simulink model "testing"  (R2022b)
settings: Solver=VariableStepAuto  StartTime=0.0  StopTime=10.0  RelTol=1e-3
values from neighbouring files (symbols this model uses):
  A = 2    [scattering_params.m]    (also in scattering_params_force_pos.m = 3; scattering_params_pos_pos.m = 1)
  b = 1    [scattering_params.m]    (also in scattering_params_force_pos.m = 40; scattering_params_pos_pos.m = 100)
  Be = 100    [scattering_params.m]    (also in scattering_params_force_pos.m; scattering_params_pos_pos.m)
  Bh = 1.5    [scattering_params.m]    (also in scattering_params_force_pos.m = 1; scattering_params_pos_pos.m = 1)
  Bm = 20*0.8    (= 16)    [scattering_params.m]
  Bs = 80    [scattering_params.m]    (also in scattering_params_force_pos.m = 10)
  Dh = 0.1    [scattering_params.m]    (also in scattering_params_force_pos.m = 16; scattering_params_pos_pos.m = 16)
  Fc = 1    [scattering_params.m]    (also in scattering_params_force_pos.m = 0.25; scattering_params_pos_pos.m = 0.25)
  Flp = 5    [scattering_params.m]    (also in scattering_params_force_pos.m = 0.5; scattering_params_pos_pos.m = 0.5)
  Jh = 1    [scattering_params.m]    (also in scattering_params_force_pos.m; scattering_params_pos_pos.m)
  Ke = 200    [scattering_params.m]    (also in scattering_params_force_pos.m; scattering_params_pos_pos.m)
  Km = 10*1    (= 10)    [scattering_params.m]
  Ks = 100    [scattering_params.m]    (also in scattering_params_force_pos.m)
  Mm = 0.5    [scattering_params.m]    (also in scattering_params_force_pos.m; scattering_params_pos_pos.m)
  Ms = 2    [scattering_params.m]    (also in scattering_params_force_pos.m; scattering_params_pos_pos.m)
  Ph = 10    [scattering_params.m]    (also in scattering_params_force_pos.m; scattering_params_pos_pos.m)
  scattering_filter_freq = 10    [scattering_params.m]    (also in scattering_params_force_pos.m; scattering_params_pos_pos.m = 100)
  time_delay = 0    [scattering_params.m]
  xe = 5    [scattering_params.m]    (also in scattering_params_force_pos.m = 2; scattering_params_pos_pos.m = 2)
settings Model: Creator=Manu  LastModifiedBy=Manu

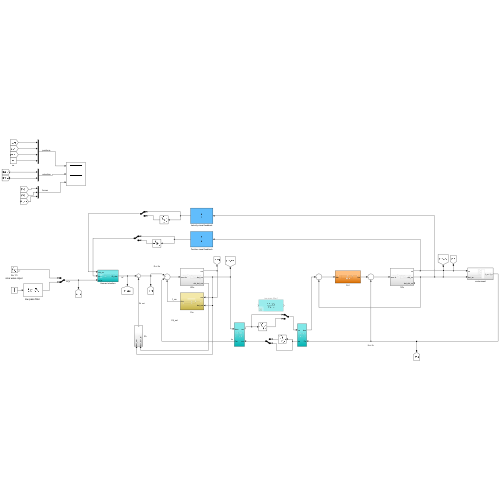
[thumbnail: Simulink's stored preview of the top-level diagram]
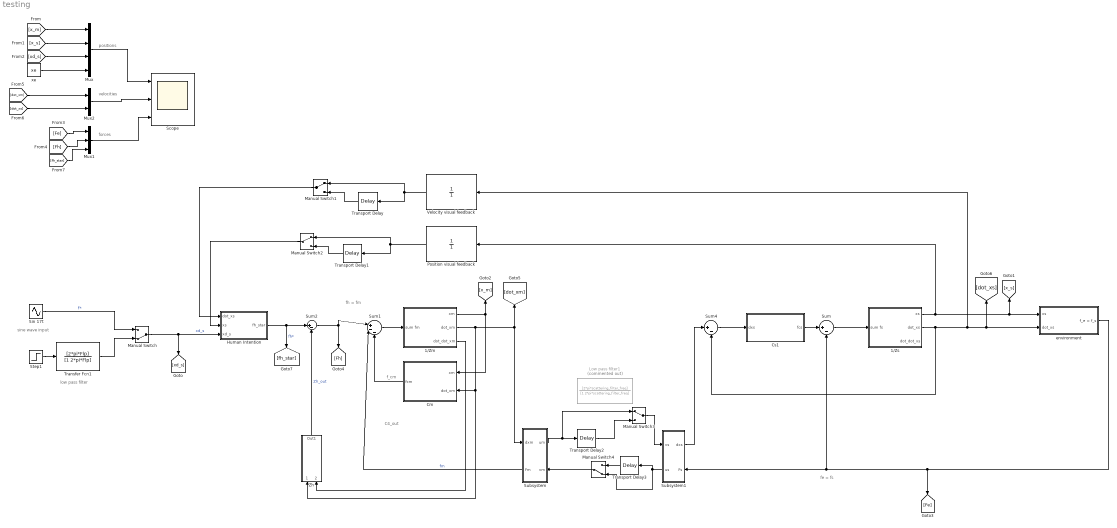
== system testing ==
  note: positions
  note: fe = fs
  note: C4_out
  note: f_cm
  note: fh = fm
  note: sine wave input
  note: low pass filter
  note: forces
  note: velocities
  1/Zm : Subsystem
  1/Zs : Subsystem
  Cm : Subsystem
  Cs1 : Subsystem
  Human Intention : Subsystem
  Low pass filter1 : TransferFcn  Commented=on  Numerator=[2*pi*scattering_filter_freq]  Denominator=[1 2*pi*scattering_filter_freq]
  Manual Switch : ManualSwitch  CurrentSetting=0
  Manual Switch1 : ManualSwitch
  Manual Switch2 : ManualSwitch
  Manual Switch3 : ManualSwitch
  Manual Switch4 : ManualSwitch  CurrentSetting=0
  Mux : Mux
  Mux1 : Mux  Inputs=3
  Mux2 : Mux  Inputs=2
  Position visual feedback : TransferFcn  Denominator=[1]
  Scope : Scope  NumInputPorts=3
  Sin 17t : Sin  Amplitude=A  Frequency=2*pi*Fc  SampleTime=0
  Step1 : Step  Time=0.5  After=A  SampleTime=0
  Subsystem : Subsystem
      settings: PortSchema="{\"entries\":[{\"content\":{\"sides\":[{\"content\":{\"connectorIds\":[\"In1\",\"Out2\"]},\"type\":\"ConnectorPlacement.EquallySpacedRectSide\",\"uuid\":\"82be490b-f4e1-4469-8bd6-488a0e070f91\"},{\"content\":{\"connectorIds\":[\"Out1\",\"In2\"],\"side\":\"RIGHT\"},\"type\":\"ConnectorPlacement.EquallySpacedRectSide\",\"uuid\":\"c4a13bf6-21c5-475e-be70-cb3636e820b8\"},{\"content\":{\"connectorIds\":[],\"side\":\"TOP\"},\"type\":\"ConnectorPlacement.EquallySpacedRectSide\",\"uuid\":\"239945ea-98d9-43ca-9337-d0acd489fa2c\"},{\"content\":{\"connectorIds\":[],\"side\":\"HIDDEN\"},\"type\":\"ConnectorPlacement.EquallySpacedRectSide\",\"uuid\":\"ab55d6c9-2d6b-496a-b62d-f74546630c92\"}]},\"type\":\"ConnectorPlacement.EquallySpacedConnector\",\"uuid\":\"f2ee4140-76ed-4153-9f7f-3580e67d072a\"}],\"packageUris\":[\"http://schema.mathworks.com/mf0/Connector/R2020b\"],\"version\":\"1.0\"}"
  Subsystem1 : Subsystem
      settings: PortSchema="{\"entries\":[{\"content\":{\"sides\":[{\"content\":{\"connectorIds\":[\"In1\",\"Out2\"]},\"type\":\"ConnectorPlacement.EquallySpacedRectSide\",\"uuid\":\"82be490b-f4e1-4469-8bd6-488a0e070f91\"},{\"content\":{\"connectorIds\":[\"Out1\",\"In2\"],\"side\":\"RIGHT\"},\"type\":\"ConnectorPlacement.EquallySpacedRectSide\",\"uuid\":\"c4a13bf6-21c5-475e-be70-cb3636e820b8\"},{\"content\":{\"connectorIds\":[],\"side\":\"TOP\"},\"type\":\"ConnectorPlacement.EquallySpacedRectSide\",\"uuid\":\"239945ea-98d9-43ca-9337-d0acd489fa2c\"},{\"content\":{\"connectorIds\":[],\"side\":\"HIDDEN\"},\"type\":\"ConnectorPlacement.EquallySpacedRectSide\",\"uuid\":\"ab55d6c9-2d6b-496a-b62d-f74546630c92\"}]},\"type\":\"ConnectorPlacement.EquallySpacedConnector\",\"uuid\":\"f2ee4140-76ed-4153-9f7f-3580e67d072a\"}],\"packageUris\":[\"http://schema.mathworks.com/mf0/Connector/R2020b\"],\"version\":\"1.0\"}"
  Sum : Sum  Inputs=|+-
  Sum1 : Sum  Inputs=|+--
  Sum2 : Sum  Inputs=|+-
  Sum4 : Sum  Inputs=|+-
  Transfer Fcn1 : TransferFcn  Numerator=[2*pi*Flp]  Denominator=[1 2*pi*Flp]
  Transport Delay{,1..3} (4 alike) : TransportDelay  DelayTime=time_delay
  Velocity visual feedback : TransferFcn  Denominator=[1]
  Zh : Subsystem
  environment : Subsystem
  xe : Constant  Value=xe
  wires:
  1/Zm/1(xm) -> Cm/1(xm), [x_m]
  Manual Switch/1 -> [xd_s], Human Intention/3(xd_s)  "xd_s"
  Zh/1(Out1) -> Sum2/2  "Zh_out"
  Sin 17t/1 -> Manual Switch/1  "F*"
  1/Zm/3(dot_dot_xm) -> Zh/2(dot_dot_xm)
  Human Intention/1(fh_star) -> Sum2/1, [fh_star]  "fh*"
  Transfer Fcn1/1 -> Manual Switch/2
  Step1/1 -> Transfer Fcn1/1
  Sum2/1 -> Sum1/1, [Fh]
  Sum1/1 -> 1/Zm/1(sum fm)
  Sum/1 -> 1/Zs/1(sum fs)
  1/Zs/2(dot_xs) -> Sum4/2, Velocity visual feedback/1, [dot_xs], environment/2(dot_xs)
  1/Zs/1(xs) -> [x_s], environment/1(xs), Position visual feedback/1
  environment/1(f_e = f_s) -> [Fe], Subsystem1/2(Fs), Sum/2
  Mux/1 -> Scope/1
  [x_s] -> Mux/2
  [xd_s] -> Mux/3
  xe/1 -> Mux/4
  [x_m] -> Mux/1
  Mux1/1 -> Scope/3
  [Fe] -> Mux1/1
  [Fh] -> Mux1/2
  [dot_xs] -> Mux2/2
  [dot_xm] -> Mux2/1
  Mux2/1 -> Scope/2
  [fh_star] -> Mux1/3
  Transport Delay1/1 -> Manual Switch2/2
  Position visual feedback/1 -> Transport Delay1/1, Manual Switch2/1
  Manual Switch2/1 -> Human Intention/2(xs)
  Subsystem/1(um) -> Transport Delay2/1, Manual Switch3/1
  Subsystem1/2(us) -> Manual Switch4/2, Transport Delay3/1
  1/Zm/2(dot_xm) -> Subsystem/1(dxm), [dot_xm], Cm/2(dot_xm), Zh/1(dot_xm)
  Subsystem/2(Fm) -> Sum1/2  "fm"
  Cm/1(fcm) -> Sum1/3
  Subsystem1/1(dxs) -> Sum4/1
  Sum4/1 -> Cs1/1(dxs)
  Cs1/1(fcs) -> Sum/1
  Manual Switch1/1 -> Human Intention/1(dot_xs)
  Transport Delay/1 -> Manual Switch1/2
  Velocity visual feedback/1 -> Transport Delay/1, Manual Switch1/1
  Transport Delay2/1 -> Manual Switch3/2
  Manual Switch3/1 -> Subsystem1/1(vs)
  Transport Delay3/1 -> Manual Switch4/1
  Manual Switch4/1 -> Subsystem/2(vm)

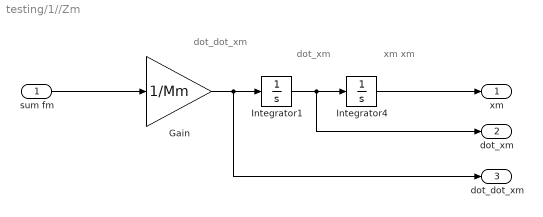
== system testing/1//Zm ==
  note: dot_dot_xm
  note: dot_xm
  note: xm
      | xm
  sum fm : Inport
  Gain : Gain  Gain=1/Mm
  Integrator1 : Integrator
  Integrator4 : Integrator
  xm : Outport
  dot_xm : Outport  Port=2
  dot_dot_xm : Outport  Port=3
  wires:
  sum fm/1 -> Gain/1
  Gain/1 -> dot_dot_xm/1, Integrator1/1
  Integrator4/1 -> xm/1
  Integrator1/1 -> dot_xm/1, Integrator4/1

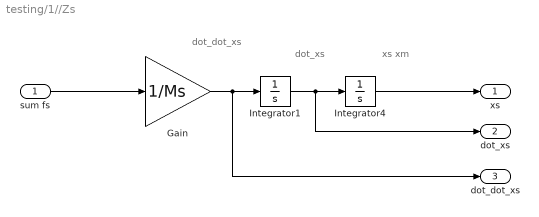
== system testing/1//Zs ==
  note: dot_dot_xs
  note: dot_xs
  note: xs
      | xm
  sum fs : Inport
  Gain : Gain  Gain=1/Ms
  Integrator1 : Integrator
  Integrator4 : Integrator
  xs : Outport
  dot_xs : Outport  Port=2
  dot_dot_xs : Outport  Port=3
  wires:
  sum fs/1 -> Gain/1
  Gain/1 -> dot_dot_xs/1, Integrator1/1
  Integrator4/1 -> xs/1
  Integrator1/1 -> dot_xs/1, Integrator4/1

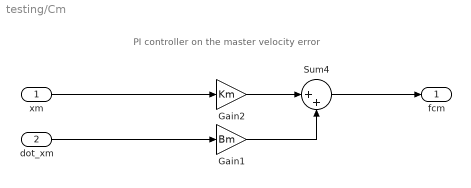
== system testing/Cm ==
  note: PI controller on the master velocity error
  xm : Inport
  dot_xm : Inport  Port=2
  Gain1 : Gain  Gain=Bm
  Gain2 : Gain  Gain=Km
  Sum4 : Sum  Inputs=|++
  fcm : Outport
  wires:
  Sum4/1 -> fcm/1
  xm/1 -> Gain2/1
  Gain2/1 -> Sum4/1
  dot_xm/1 -> Gain1/1
  Gain1/1 -> Sum4/2

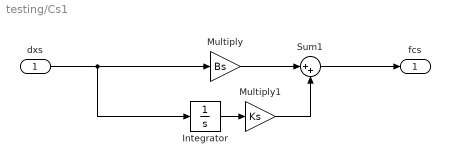
== system testing/Cs1 ==
  dxs : Inport
  Integrator : Integrator
  Multiply : Gain  Gain=Bs
  Multiply1 : Gain  Gain=Ks
  Sum1 : Sum  Inputs=|++
  fcs : Outport
  wires:
  dxs/1 -> Integrator/1, Multiply/1
  Multiply1/1 -> Sum1/2
  Multiply/1 -> Sum1/1
  Sum1/1 -> fcs/1
  Integrator/1 -> Multiply1/1

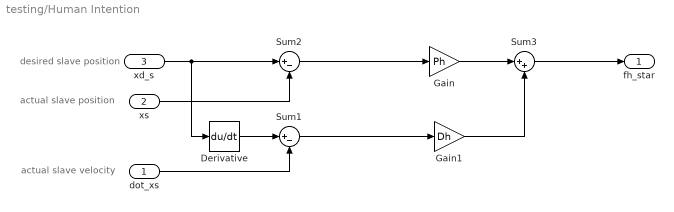
== system testing/Human Intention ==
  note: actual slave velocity
  note: actual slave position
  note: desired slave position
  dot_xs : Inport
  xs : Inport  Port=2
  xd_s : Inport  Port=3
  Derivative : Derivative
  Gain : Gain  Gain=Ph
  Gain1 : Gain  Gain=Dh
  Sum1 : Sum  Inputs=|+-
  Sum2 : Sum  Inputs=|+-
  Sum3 : Sum  Inputs=|++
  fh_star : Outport
  wires:
  xs/1 -> Sum2/2
  dot_xs/1 -> Sum1/2
  Sum2/1 -> Gain/1
  Sum1/1 -> Gain1/1
  Gain1/1 -> Sum3/2
  Gain/1 -> Sum3/1
  Sum3/1 -> fh_star/1
  xd_s/1 -> Derivative/1, Sum2/1
  Derivative/1 -> Sum1/1

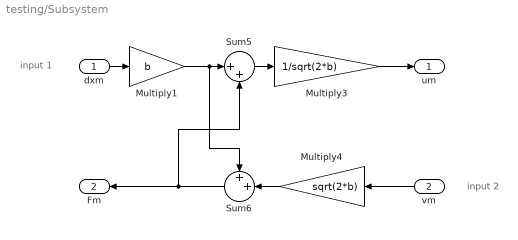
== system testing/Subsystem ==
  note: input 2
  note: input 1
  dxm : Inport
  vm : Inport  Port=2
  Multiply1 : Gain  Gain=b
  Multiply3 : Gain  Gain=1/sqrt(2*b)
  Multiply4 : Gain  Gain=sqrt(2*b)
  Sum5 : Sum  Inputs=|++
  Sum6 : Sum  Inputs=++|
  um : Outport
  Fm : Outport  Port=2
  wires:
  Sum6/1 -> Fm/1, Sum5/2
  Multiply1/1 -> Sum6/1, Sum5/1
  Sum5/1 -> Multiply3/1
  Multiply4/1 -> Sum6/2
  vm/1 -> Multiply4/1
  Multiply3/1 -> um/1
  dxm/1 -> Multiply1/1

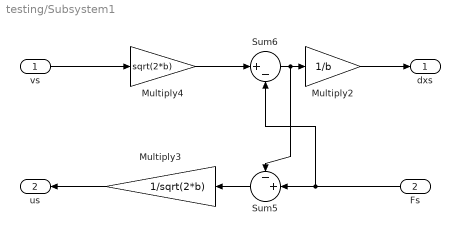
== system testing/Subsystem1 ==
  vs : Inport
  Fs : Inport  Port=2
  Multiply2 : Gain  Gain=1/b
  Multiply3 : Gain  Gain=1/sqrt(2*b)
  Multiply4 : Gain  Gain=sqrt(2*b)
  Sum5 : Sum  Inputs=-+|
  Sum6 : Sum  Inputs=|+-
  dxs : Outport
  us : Outport  Port=2
  wires:
  Sum6/1 -> Sum5/1, Multiply2/1
  Sum5/1 -> Multiply3/1
  Fs/1 -> Sum5/2, Sum6/2
  vs/1 -> Multiply4/1
  Multiply2/1 -> dxs/1
  Multiply3/1 -> us/1
  Multiply4/1 -> Sum6/1

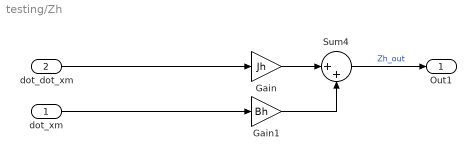
== system testing/Zh ==
  dot_xm : Inport
  dot_dot_xm : Inport  Port=2
  Gain : Gain  Gain=Jh
  Gain1 : Gain  Gain=Bh
  Sum4 : Sum  Inputs=|++
  Out1 : Outport
  wires:
  dot_dot_xm/1 -> Gain/1
  Gain1/1 -> Sum4/2
  Gain/1 -> Sum4/1
  Sum4/1 -> Out1/1  "Zh_out"
  dot_xm/1 -> Gain1/1

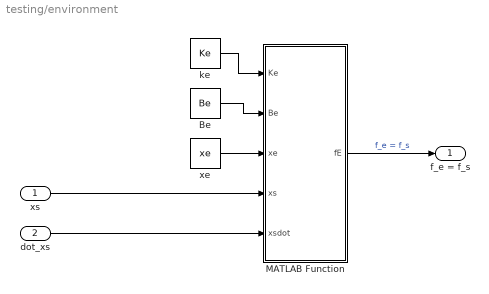
== system testing/environment ==
  xs : Inport
  dot_xs : Inport  Port=2
  Be : Constant  Value=Be
  MATLAB Function : MATLAB Function  TreatAsAtomicUnit=on
  ke : Constant  Value=Ke
  xe : Constant  Value=xe
  f_e = f_s : Outport
  wires:
  MATLAB Function/1(fE) -> f_e = f_s/1  "f_e = f_s"
  xs/1 -> MATLAB Function/4(xs)
  xe/1 -> MATLAB Function/3(xe)
  dot_xs/1 -> MATLAB Function/5(xsdot)
  ke/1 -> MATLAB Function/1(Ke)
  Be/1 -> MATLAB Function/2(Be)

== matlab function testing/environment/MATLAB Function ==
  data: Ke input; fE output; Be input; xe input; xs input; xsdot input
function fE = environment(Ke, Be, xe, xs, xsdot)
    if xs > xe
        fE = Ke * (xs - xe) + Be * xsdot; % Plot both contributions Ke and Be
    else
        fE = 0;
    end
end
